simulink model "robot_model_wro"  (R2024b)
settings: Solver=VariableStepAuto  StartTime=0.0  StopTime=10.0  RelTol=1e-3  EnableMultiTasking=on
libraries: slpidlib x1
settings Model: Creator=ahmed  LastModifiedBy=ahmed
settings SolverCC: PositivePriorityOrder=on
settings DataIOCC: InspectSignalLogs=on
settings OptimizationCC: DefaultParameterBehavior=Inlined  EnhancedBackFolding=on  PassReuseOutputArgsAs=Individual arguments  ZeroExternalMemoryAtStartup=off  ZeroInternalMemoryAtStartup=off  MaxStackSize=64  OptimizeBlockOrder=speed  DifferentSizesBufferReuse=on  EfficientTunableParamExpr=on
settings DebuggingCC: ParameterTunabilityLossMsg=error
settings HardwareCC: ProdBitPerPointer=32  ProdBitPerSizeT=32  ProdBitPerPtrDiffT=32  ProdLargestAtomicFloat=None  ProdWordSize=32  ProdHWDeviceType=Custom Processor->Custom
settings ModelReferenceCC: ModelReferenceNumInstancesAllowed=Single
settings SFSimCC: MATLABDynamicMemAlloc=off
settings RTWCC: Description=Embedded Coder  SystemTargetFile=ert.tlc  TemplateMakefile=ert_default_tmf
settings CodeAppCC: ForceParamTrailComments=on  IgnoreCustomStorageClasses=off  OperatorAnnotations=on  SimulinkDataObjDesc=on  SFDataObjDesc=on  InsertBlockDesc=on
settings ERTTargetCC: ERTCustomFileTemplate=example_file_process.tlc

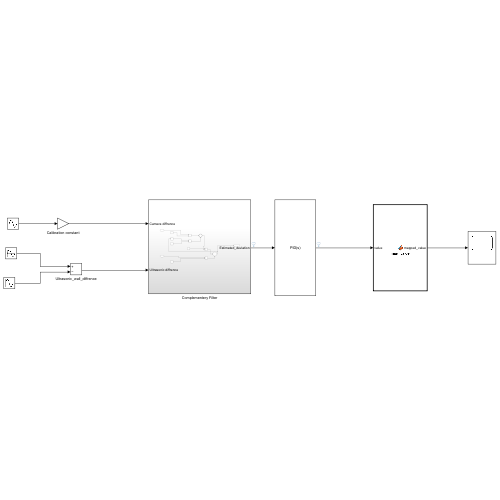
[thumbnail: Simulink's stored preview of the top-level diagram]
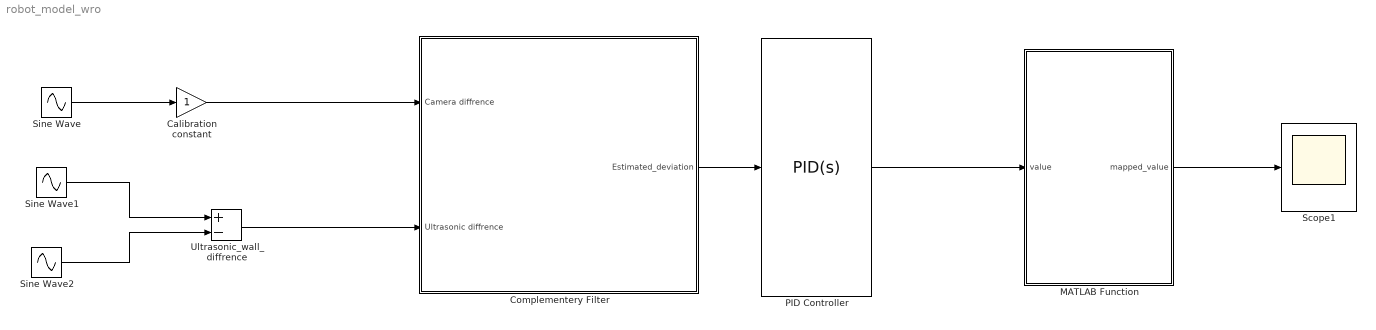
== system robot_model_wro ==
  Calibration constant : Gain
  Complementery Filter : Subsystem
  MATLAB Function : MATLAB Function  TreatAsAtomicUnit=on
  PID Controller : slpidlib/PID Controller  Controller=PID  Form=Parallel  TimeDomain=Continuous-time  UseExternalTs=off  SampleTime=-1  IntegratorMethod=Forward Euler  FilterMethod=Forward Euler  ControllerParametersSource=internal  P=1.3426  I=0.2335  UseKiTs=off  D=0.1442  UseExternalDerivativeSource=off  N=100  UseFilter=on  TunerSelectOption=Transfer Function Based (PID Tuner App)  InitialConditionSource=internal  InitialConditionForIntegrator=0  InitialConditionForFilter=0  DifferentiatorICPrevScaledInput=0  ExternalReset=none  TrackingMode=off  Kt=1  LimitOutput=off  SatLimitsSource=internal  UpperSaturationLimit=inf  LowerSaturationLimit=-inf  LinearizeAsGain=on  AntiWindupMode=none  Kb=1  LimitIntegrator=off  UpperIntegratorSaturationLimit=inf  LowerIntegratorSaturationLimit=-inf  POutMin=[]  POutMax=[]  IOutMin=[]  IOutMax=[]  DOutMin=[]  DOutMax=[]  NOutMin=[]  NOutMax=[]  SumOutMin=[]  SumOutMax=[]  SaturationOutMin=[]  SaturationOutMax=[]  PParamMin=[]  PParamMax=[]  IParamMin=[]  IParamMax=[]  DParamMin=[]  DParamMax=[]  NParamMin=[]  NParamMax=[]  KbParamMin=[]  KbParamMax=[]  KtParamMin=[]  KtParamMax=[]  KbOutMin=[]  KbOutMax=[]  KtOutMin=[]  KtOutMax=[]  IntegratorOutMin=[]  IntegratorOutMax=[]  FilterOutMin=[]  FilterOutMax=[]  SumI1OutMin=[]  SumI1OutMax=[]  SumI2OutMin=[]  SumI2OutMax=[]  SumI3OutMin=[]  SumI3OutMax=[]  SumI4OutMin=[]  SumI4OutMax=[]  SumDOutMin=[]  SumDOutMax=[]  DifferentiatorOutMin=[]  DifferentiatorOutMax=[]  FilterDiffOutCoefMin=[]  FilterDiffOutCoefMax=[]  ReciprocalOutMin=[]  ReciprocalOutMax=[]  SumDenOutMin=[]  SumDenOutMax=[]  SumNumOutMin=[]  SumNumOutMax=[]  DivideOutMin=[]  DivideOutMax=[]  UdiffTsProdOutMin=[]  UdiffTsProdOutMax=[]  NTsProdOutMin=[]  NTsProdOutMax=[]  UintegralTsProdOutMin=[]  UintegralTsProdOutMax=[]  UngainTsProdOutMin=[]  UngainTsProdOutMax=[]  ClampingZeroOutDataTypeStr=Inherit: Inherit via back propagation  ClampingZeroOutMin=[]  ClampingZeroOutMax=[]  FilterDenConstantOutDataTypeStr=Inherit: Inherit via back propagation  FilterDenConstantOutMin=[]  FilterDenConstantOutMax=[]  PCopyOutDataTypeStr=Inherit: Inherit via back propagation  PCopyOutMin=[]  PCopyOutMax=[]  NCopyOutDataTypeStr=Inherit: Inherit via back propagation  NCopyOutMin=[]  NCopyOutMax=[]  IntegratorContinuousStateAttributes=''  IntegratorStateMustResolveToSignalObject=off  IntegratorRTWStateStorageClass=Auto  FilterContinuousStateAttributes=''  FilterStateMustResolveToSignalObject=off  FilterRTWStateStorageClass=Auto  ParallelPVariant=InternalParameters  IdealPVariant=Disabled  IVariant=InternalParameters  DVariant=InternalParameters  IntegratorVariant=Continuous  SatVariant=Disabled  AWVariant=Passthrough  PCopyVariant=Disabled  TRVariant=Disabled  FdbkBlocksVariant=Forward  IdealPFdbkVariant=Disabled  SatFdbkVariant=Disabled  DerivativeFilterVariant=ContFilter  NVariant=InternalParameters  NCopyVariant=Disabled  FilterICVariant=InternalICsFilter  IntegratorICVariant=InternalICs  ExternalResetVariant=Disabled  TRSumVariant=Passthrough  SumFdbkVariant=Disabled  SumVariant=Sum_PID  TsampFilterVariant=InternalTs  TsampNgainVariant=Passthrough  TsampIntegralVariant=Disabled_SignalSpec  ExternalSaturationOutDataTypeStr=Inherit: Same as second input  DerivativeSourceVariant=ErrorSignal  PreIntVariant=InternalPreInt
  Scope1 : Scope
  Sine Wave : Sin  Amplitude=25  SampleTime=0
  Sine Wave1 : Sin  Amplitude=25  SampleTime=0
  Sine Wave2 : Sin  Amplitude=25  SampleTime=0
  Ultrasonic_wall_diffrence : Sum  Inputs=+-
  wires:
  Sine Wave1/1 -> Ultrasonic_wall_diffrence/1
  Sine Wave2/1 -> Ultrasonic_wall_diffrence/2
  Sine Wave/1 -> Calibration constant/1
  Ultrasonic_wall_diffrence/1 -> Complementery Filter/2(Ultrasonic diffrence)
  Calibration constant/1 -> Complementery Filter/1(Camera diffrence)
  Complementery Filter/1(Estimated_deviation) -> PID Controller/1
  PID Controller/1 -> MATLAB Function/1(value)
  MATLAB Function/1(mapped_value) -> Scope1/1

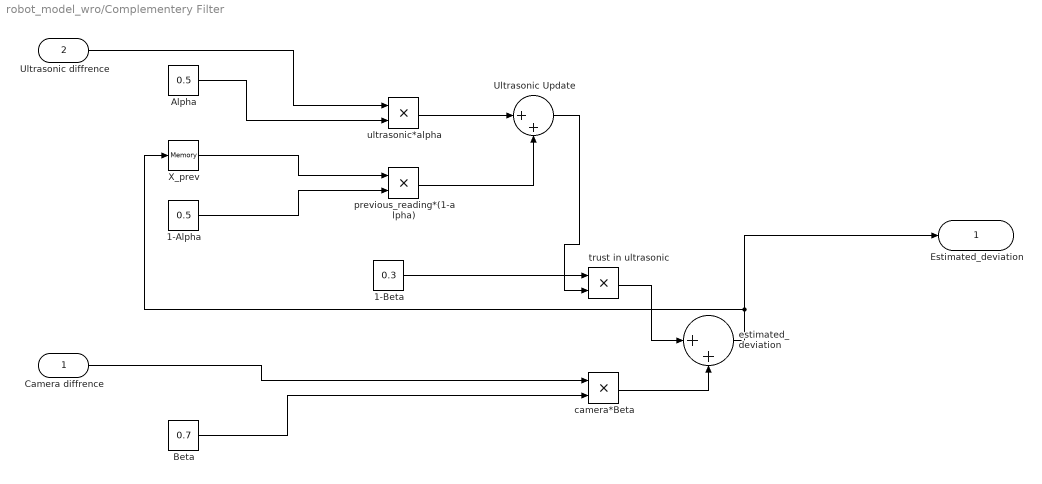
== system robot_model_wro/Complementery Filter ==
  Camera diffrence : Inport
  Ultrasonic diffrence : Inport  Port=2
  1-Alpha : Constant  Value=0.5
  1-Beta : Constant  Value=0.3
  Alpha : Constant  Value=0.5
  Beta : Constant  Value=0.7
  Ultrasonic Update : Sum  Inputs=|++
  X_prev : Memory
  camera*Beta : Product
  estimated_deviation : Sum  Inputs=|++
  previous_reading*(1-alpha) : Product
  trust in ultrasonic : Product
  ultrasonic*alpha : Product
  Estimated_deviation : Outport
  wires:
  Ultrasonic diffrence/1 -> ultrasonic*alpha/1
  Alpha/1 -> ultrasonic*alpha/2
  1-Alpha/1 -> previous_reading*(1-alpha)/2
  X_prev/1 -> previous_reading*(1-alpha)/1
  ultrasonic*alpha/1 -> Ultrasonic Update/1
  previous_reading*(1-alpha)/1 -> Ultrasonic Update/2
  Camera diffrence/1 -> camera*Beta/1
  Beta/1 -> camera*Beta/2
  1-Beta/1 -> trust in ultrasonic/1
  Ultrasonic Update/1 -> trust in ultrasonic/2
  camera*Beta/1 -> estimated_deviation/2
  trust in ultrasonic/1 -> estimated_deviation/1
  estimated_deviation/1 -> X_prev/1, Estimated_deviation/1

== matlab function robot_model_wro/MATLAB Function ==
  data: value input; mapped_value output
function mapped_value = map_value(value)
%MAP_VALUE maps a value from one range to another

    from_low=-50;
    from_high= 50;
    to_low=30;
    to_high=160;
    % Avoid division by zero
    if (from_high - from_low) == 0
        mapped_value = to_low;
        return;
    end

    % mapping equation
    mapped_value = (value - from_low) / (from_high - from_low) * ...
                   (to_high - to_low) + to_low;
end
